simulink model "Mass_Damper"  (R2020b)
settings: Solver=VariableStepAuto  StartTime=0.0  StopTime=T_var  MaxStep=0.001  RelTol=1e-3
values from neighbouring files (symbols this model uses):
  b = 5    [damper.m]    (also in transferf.m)
  F = 10    [damper.m]    (also in transferf.m = 1)
  k = 20    [damper.m]    (also in transferf.m)
  M = 10    [damper.m]    (also in transferf.m)
settings Model: Creator=Raihan mahmud  LastModifiedBy=Raihan mahmud

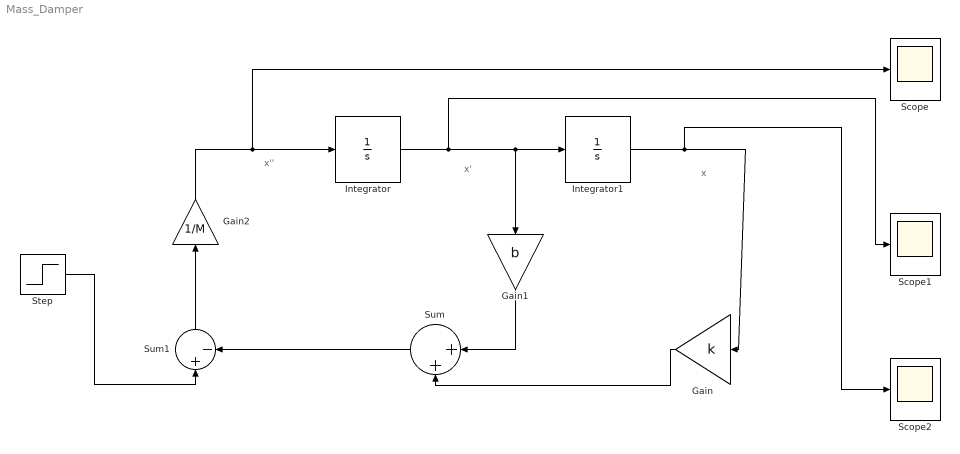
== system Mass_Damper ==
  note: x
  note: x'
  note: x''
  Gain : Gain  Gain=k
  Gain1 : Gain  Gain=b
  Gain2 : Gain  Gain=1/M
  Integrator : Integrator
  Integrator1 : Integrator
  Scope : Scope
  Scope1 : Scope
  Scope2 : Scope
  Step : Step  After=F  SampleTime=0
  Sum : Sum  Inputs=|++
  Sum1 : Sum  Inputs=|+-
  wires:
  Gain2/1 -> Scope/1, Integrator/1
  Gain1/1 -> Sum/1
  Gain/1 -> Sum/2
  Step/1 -> Sum1/1
  Sum/1 -> Sum1/2
  Sum1/1 -> Gain2/1
  Integrator/1 -> Integrator1/1, Gain1/1, Scope1/1
  Integrator1/1 -> Scope2/1, Gain/1
